simulink library "hdlNFPMathLib"  (R2019a)
settings: Solver=VariableStepAuto  StartTime=0.0  StopTime=10.0  RelTol=1e-3
libraries: simulink x3, hdlcoderNFPCast x2
settings Model: Creator=The MathWorks, Inc.  LastModifiedBy=The MathWorks, Inc.
settings DataIOCC: ReturnWorkspaceOutputs=off
settings DebuggingCC: ArithmeticOperatorsInVariantConditions=warning
settings SFSimCC: SimUseLocalCustomCode=off
settings RTWCC: RTWUseLocalCustomCode=off
settings CodeAppCC: StateflowObjectComments=on

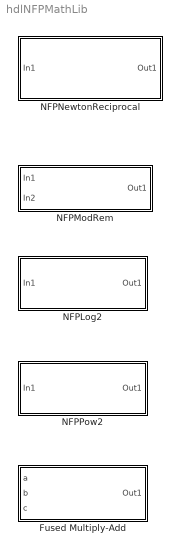
== system hdlNFPMathLib ==
  Fused Multiply-Add : Subsystem  mask(Fused Multiply-Add){FMA=on}
      mask prompts: FMA "Floating-point fused multiply-add"
      mask help: Performing fused multiply-add (FMA) operations on single inputs.
      mask init:
      | FMAstr = get_param(gcb, 'FMA');
      | if strcmp(FMAstr, 'on')
      |     fused = true;
      | else
      |     fused = false;
      | end
      mask Display:
      | port_label('input', 1, 'a');
      | port_label('input', 2, 'b');
      | port_label('input', 3, 'c');
      | 
      | FMAstr = get_param(gcb, 'FMA');
      | 
      | if strcmp(FMAstr, 'on')
      |     disp('c + (a.*b)\n\n(fused)');
      | else
      |     disp('c + (a.*b)');
      | end
  NFPLog2 : Subsystem
  NFPModRem : Subsystem  VariantControl=Variant1  mask{MAX_ITERATIONS=0, ModOrRem=Rem, MaxIterations=32, ModOrRemText=0}
      mask prompts: MAX_ITERATIONS "NumberOfIterations"; ModOrRem "Function"
      mask init:
      | if (ModOrRem == 1)
      |     ModOrRemText = 'Rem';
      | else
      |     ModOrRemText = 'Mod';
      | end
      | 
      | if (MaxIterations == 1)
      |     MAX_ITERATIONS = 32;
      | elseif (MaxIterations == 2)
      |     MAX_ITERATIONS = 64;
      | else
      |     MAX_ITERATIONS = 128;
      | end
      mask TypeOptions ModOrRem: Rem | Mod
      mask TypeOptions MaxIterations: 32 | 64 | 128
      mask Display: disp(ModOrRemText)
  NFPNewtonReciprocal : Subsystem  mask(NFP Newton Raphson Reciprocal){NumberOfIterations=3, SampleTime=-1}
      mask prompts: NumberOfIterations "Number Of Iterations"
      mask help:
      | For floating-point datatype, this block uses fixed-point arithmetics in each NR iteration while 'HDL Reciprocal' block uses floating-point arithmetics.
      |
      | Fixed-point datatype is not supported with this block.
      mask init:
      | numIters = NumberOfIterations;
  NFPPow2 : Subsystem

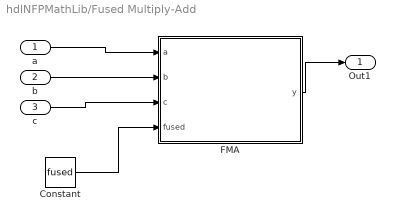
== system hdlNFPMathLib/Fused Multiply-Add ==
  a : Inport
  b : Inport  Port=2
  c : Inport  Port=3
  Constant : Constant  Value=fused  SampleTime=-1
  FMA : MATLAB Function  TreatAsAtomicUnit=on  mask{Function=0}
      mask init:
      | Function = 'pow2';
  Out1 : Outport
  wires:
  a/1 -> FMA/1(a)
  FMA/1(y) -> Out1/1
  b/1 -> FMA/2(b)
  c/1 -> FMA/3(c)
  Constant/1 -> FMA/4(fused)

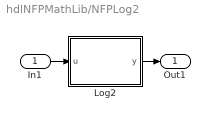
== system hdlNFPMathLib/NFPLog2 ==
  In1 : Inport
  Log2 : MATLAB Function  TreatAsAtomicUnit=on  mask{Function=0}
      mask init:
      | Function = 'log2';
  Out1 : Outport
  wires:
  In1/1 -> Log2/1(u)
  Log2/1(y) -> Out1/1

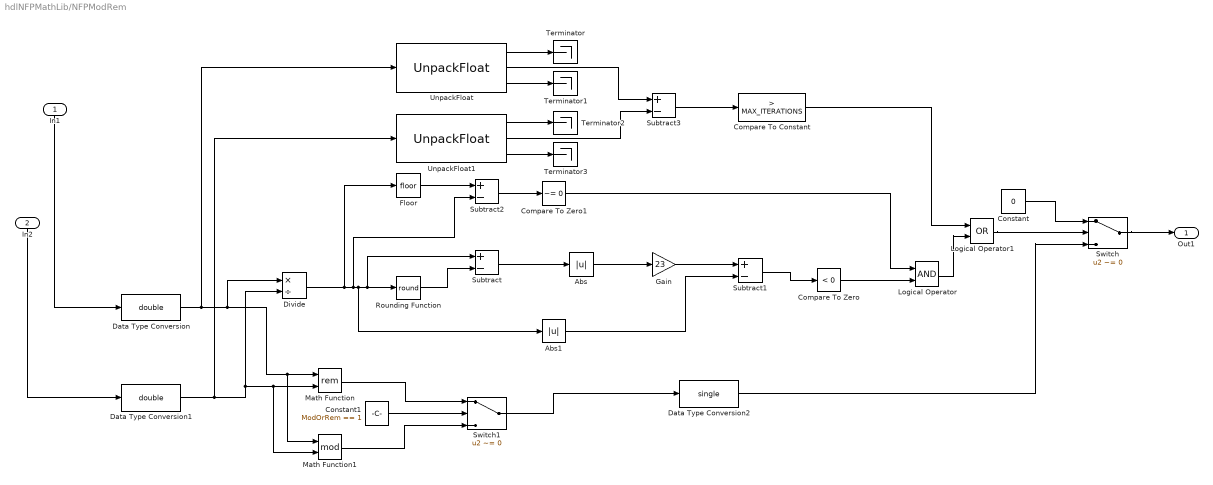
== system hdlNFPMathLib/NFPModRem ==
  In1 : Inport
  In2 : Inport  Port=2
  Abs : Abs
  Abs1 : Abs
  Compare To Constant : simulink/Logic and Bit Operations/Compare To Constant  relop=>  const=MAX_ITERATIONS  OutDataTypeStr=boolean
  Compare To Zero : simulink/Logic and Bit Operations/Compare To Zero  relop=<  OutDataTypeStr=boolean
  Compare To Zero1 : simulink/Logic and Bit Operations/Compare To Zero  relop=~=  OutDataTypeStr=boolean
  Constant : Constant  Value=0  OutDataTypeStr=single  SampleTime=-1
  Constant1 : Constant  Value=ModOrRem == 1  SampleTime=-1
  Data Type Conversion : DataTypeConversion  OutDataTypeStr=double
  Data Type Conversion1 : DataTypeConversion  OutDataTypeStr=double
  Data Type Conversion2 : DataTypeConversion  OutDataTypeStr=single
  Divide : Product  Inputs=*/  SaturateOnIntegerOverflow=on  RndMeth=Zero
  Floor : Rounding
  Gain : Gain  Gain=23
  Logical Operator : Logic  AllPortsSameDT=off  OutDataTypeStr=boolean
  Logical Operator1 : Logic  Operator=OR  AllPortsSameDT=off  OutDataTypeStr=boolean
  Math Function : Math  Operator=rem  SaturateOnIntegerOverflow=on
  Math Function1 : Math  Operator=mod  SaturateOnIntegerOverflow=on
  Rounding Function : Rounding  Operator=round
  Subtract : Sum  Inputs=+-
  Subtract1 : Sum  Inputs=+-
  Subtract2 : Sum  Inputs=+-
  Subtract3 : Sum  Inputs=+-  AccumDataTypeStr=int16  OutDataTypeStr=int16  SaturateOnIntegerOverflow=on
  Switch : Switch  Criteria=u2 ~= 0
  Switch1 : Switch  Criteria=u2 ~= 0
  Terminator{,1..3} (4 alike) : Terminator
  UnpackFloat : hdlcoderNFPCast/UnpackFloat  dataType=double
      settings: SourceProductName=Simulink  SourceProductBaseCode=SL
  UnpackFloat1 : hdlcoderNFPCast/UnpackFloat  dataType=double
      settings: SourceProductName=Simulink  SourceProductBaseCode=SL
  Out1 : Outport
  wires:
  In1/1 -> Data Type Conversion/1
  In2/1 -> Data Type Conversion1/1
  Data Type Conversion1/1 -> UnpackFloat1/1, Math Function1/2, Math Function/2, Divide/2
  Data Type Conversion/1 -> UnpackFloat/1, Math Function1/1, Math Function/1, Divide/1
  Data Type Conversion2/1 -> Switch/3
  Subtract/1 -> Abs/1
  Rounding Function/1 -> Subtract/2
  Divide/1 -> Floor/1, Subtract2/2, Abs1/1, Subtract/1, Rounding Function/1
  Abs/1 -> Gain/1
  Gain/1 -> Subtract1/1
  Abs1/1 -> Subtract1/2
  Compare To Zero/1 -> Logical Operator/2
  Subtract1/1 -> Compare To Zero/1
  Switch/1 -> Out1/1
  Constant/1 -> Switch/1
  Floor/1 -> Subtract2/1
  Subtract2/1 -> Compare To Zero1/1
  Logical Operator1/1 -> Switch/2
  Compare To Zero1/1 -> Logical Operator/1
  UnpackFloat/1 -> Terminator/1
  UnpackFloat/3 -> Terminator1/1
  UnpackFloat1/3 -> Terminator3/1
  UnpackFloat1/1 -> Terminator2/1
  UnpackFloat/2 -> Subtract3/1
  UnpackFloat1/2 -> Subtract3/2
  Subtract3/1 -> Compare To Constant/1
  Logical Operator/1 -> Logical Operator1/2
  Compare To Constant/1 -> Logical Operator1/1
  Switch1/1 -> Data Type Conversion2/1
  Math Function1/1 -> Switch1/3
  Math Function/1 -> Switch1/1
  Constant1/1 -> Switch1/2

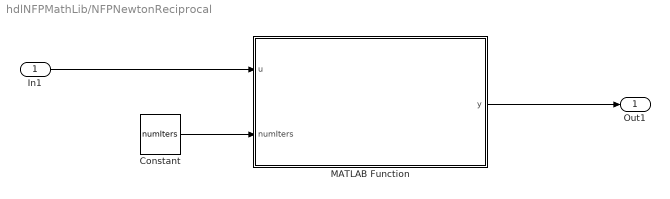
== system hdlNFPMathLib/NFPNewtonReciprocal ==
  In1 : Inport
  Constant : Constant  Value=numIters  VectorParams1D=off  OutDataTypeStr=uint8  SampleTime=-1
  MATLAB Function : MATLAB Function  TreatAsAtomicUnit=on
  Out1 : Outport
  wires:
  Constant/1 -> MATLAB Function/2(numIters)
  In1/1 -> MATLAB Function/1(u)
  MATLAB Function/1(y) -> Out1/1

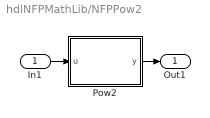
== system hdlNFPMathLib/NFPPow2 ==
  In1 : Inport
  Pow2 : MATLAB Function  TreatAsAtomicUnit=on  mask{Function=0}
      mask init:
      | Function = 'pow2';
  Out1 : Outport
  wires:
  Pow2/1(y) -> Out1/1
  In1/1 -> Pow2/1(u)

== matlab function hdlNFPMathLib/NFPLog2/Log2 ==
  data: u input; y output
function y = LOG2(u)
%#codegen
    u = double(u);
    y = zeros(size(u), 'single');
    
    for ii = 1:1:numel(u)
        if (u(ii) < 0)
            y(ii) = single(NaN);
        else
            y(ii) = single(log(u(ii))/log(2));
        end
    end
end

== matlab function hdlNFPMathLib/NFPNewtonReciprocal/MATLAB Function ==
  data: u input; y output; numIters input
function y = eml_al_nr_reciprocal_v2(u,numIters)
% Algorithm Lowering Library Function for Newto-Raphson reciprocal

% Copyright 2013-2014 MathWorks,Inc.
%#codegen

% y = 1/u

coder.allowpcode('plain');
% 
% if ~isempty(coder.target)
%     eml_prefer_const(u);
%     eml_prefer_const(numIters);
% end

%Compute input argument dimensions
sz = size(u);
if isfi(u)
    outLen = numberofelements(u);
else
    outLen = numel(u);
end

% Pre-allocation and initialization

% double input
if isa(u,'double')
    y = coder.nullcopy(zeros(sz));
    uInput = double(0);     
end

% single input
if isa(u,'single')
    y = coder.nullcopy(single(zeros(sz)));
    uInput = single(0);    
end

% fixed point input
if ~isfloat(u)
    assert('Non-floating data types are not supported');
    return;
    
    [uNT,yNT,yFm] = locaGetOutputFixptAttrib(u);
    
    if (yNT.FractionLength == 0)
        switch(yNT.WordLength)
            case 8
                if yNT.SignednessBool
                    y = int8(0);
                else
                    y = uint8(0);
                end
            case 16
                if yNT.SignednessBool
                    y = int16(0);
                else
                    y = uint16(0);
                end
            case 32
                if yNT.SignednessBool
                    y = int32(0);
                else
                    y = uint32(0);
                end
            case 64
                if yNT.SignednessBool
                    y = int64(0);
                else
                    y = uint64(0);
                end
            otherwise
                y = coder.nullcopy(fi(zeros(sz),yNT));
        end
    else
        y = coder.nullcopy(fi(zeros(sz),yNT));
    end

    uInput = fi(u,uNT,yFm);
end

% Newton-Raphson Reciprocal Algorithm
for idx = 1:outLen
    u_idx = u(idx);
    
    if (u_idx < cast(0,'like',u_idx))
        uInput(:) = -u_idx;
        u_sign_change = true;
    else
        uInput(:) = u_idx;
        u_sign_change = false;
    end
    
    % Newton-Raphson kernel iterations
    if isfloat(uInput)
        % floating point
        b = reciprocal_nr_kernel(uInput,numIters);
    else
        % fixed point
        b = reciprocal_nr_kernel_fi(uInput,numIters);
    end
    
    if u_sign_change
        y(idx) = -b;
    else
        y(idx) = b;
    end
    
end

end   % function

% ------------------------------------------
% local function
% ------------------------------------------
function b  = reciprocal_nr_kernel(a,n)
% kernel to iteratively compute Newton-Raphson reciprocal
%#codegen
% 
% if ~isempty(coder.target)
%     eml_prefer_const(n);
% end

if a == cast(0,'like',a)
    b = cast(1/a,'like',a);
    return;
elseif abs(a) == cast(inf,'like',a)    
    b = cast(1/a,'like',a);    
    return;
end

f = abs(a);

[t,e] = log2(f);

b = cast(1,'like',a);

if ~isfloat(a) || isnan(a)
    for i = 1:n
        b(:) =  b*(2-b*t);
    end
else
    if strcmpi('single', class(a))
        MWL = 25; MFL = 23;
    else % double
        MWL = 25; MFL = 23;
    end
    fm = fimath(hdlfimath, 'ProductMode', 'SpecifyPrecision', ...
        'ProductWordLength', MWL, 'ProductFractionLength', MFL, ...
        'SumMode', 'SpecifyPrecision', ...
        'SumWordLength', MWL, 'SumFractionLength', MFL);
    b = fi(b, 0, MWL, MFL, fm);
    t = fi(t, 0, MWL, MFL, fm);
    x = fi(2, 0, MWL, MFL, fm);
    for i = 1:n
        b(:) =  b*(x-b*t);
    end
    b = cast(b, 'like', a);
end

b = b*pow2(-e);

end

% -----------------------------------------
% fixed-point kernel
% -----------------------------------------
function y = reciprocal_nr_kernel_fi(u,n)
%# codegen 

[a,p] = fxpFREXP(u);

isInputZero = isequal(u,cast(0,'like',u));

% if input is zero, no need to denormalize result
% since it is the max value for the output format

if isInputZero && (p > cast(0,'like',p))
    p = cast(0,'like',p);
end

localFm = u.fimath;

wl = u.WordLength;
fl = u.FractionLength;

b = fi(1,0,wl,wl-2,localFm);

for i = 1:n
    b(:) = b*(cast(2,'like',b) - b*a); 
end

if u.Signed
    extraIntLength = 1;
else
    extraIntLength = 0;
end

output_fl = (wl-fl-1-extraIntLength);

if b.WordLength > 1   
    if p >= 0  
        if isInputZero
            b = bitsra(b,extraIntLength);
        end
        
        keep_extra_bit = 1-fl-extraIntLength;    % Extra number of LSB to keep
                                                 % (before being thrown away by bitsra()),
                                                 % which is distance between fractionlength of 
                                                 % intermediate datatype and
                                                 % output datatype, which
                                                 % is equal to [output_fl - (wl-2)] 
        
        if ((keep_extra_bit >0) && ~isInputZero)
            y = reinterpretcast(bitsra(b,p-1),numerictype(false,wl,wl-1)); % keep one extra bit to have better precision
            y = fi(y,numerictype(u.Signed,wl,output_fl));
        else
            y = fi(bitsra(b,p),numerictype(u.Signed,wl,output_fl));
        end
    else
        b = reinterpretcast(b,numerictype(false,wl,0));
        y = reinterpretcast(bitsra(b,fl-1+p),numerictype(false,wl,wl-fl-1));
        y = fi(y,numerictype(u.Signed,wl,output_fl));
    end
else
    y = b;
    y = fi(y,numerictype(u.Signed,wl,output_fl));
end

end

% ----------------------------------------
% fixed point normalization function
% ----------------------------------------
function [y,r]= fxpFREXP(u)
% fxpFREXP(u): Range normalization for fixed-point
%
% This function assumes:
%
%   1) u is a POSITIVE-valued
%   2) u is a FI fixed-point binary point scaled type
%   3) 2 < u.WordLength <= 128
%
% *** The CALLER must check for this before calling fxpFREXP ***
%# codegen 

if ~isfi(u)
    error('fi:internal:mustbefi','Input must be fi.\n');
end

WL = u.WordLength;

if WL > 128
    error('fi:internal:mustlessthan128','Word Length of fi object cannot exceed 128\n');
end

if WL == 1
    v = reinterpretcast(fi(u,false,2,u.FractionLength),numerictype(false,2,0));
else
    v = reinterpretcast(u,numerictype(false,WL,0));
end

if WL > 64
    % Assuming 64< WL <= 128 
    
    % NOTE: (2^64 - 1) not representable in a double with 52-bit mantissa
    r  = bitsll(int16(v > fi(2^64-1,false,WL,0,'hex','ffffffffffffffff')), 6);
    v  = bitsra(v, r);

    sh = bitsll(int16(v > (2^32 - 1)), 5);
    v  = bitsra(v, sh);
    r  = bitor( r, sh);

    sh = bitsll(int16(v > (2^16 - 1)), 4);
    v  = bitsra(v, sh);
    r  = bitor( r, sh);

    sh = bitsll(int16(v > ( 2^8 - 1)), 3);
    v  = bitsra(v, sh);
    r  = bitor( r, sh);

    sh = bitsll(int16(v > ( 2^4 - 1)), 2);
    v  = bitsra(v, sh);
    r  = bitor( r, sh);

    sh = bitsll(int16(v > ( 2^2 - 1)), 1);
    v  = bitsra(v, sh);
    r  = bitor( r, sh);
    
    elseif WL > 32
    % Assuming 32 < WL <= 64 here
    r  = bitsll(int16(v > (2^32 - 1)), 5);
    v  = bitsra(v, r);

    sh = bitsll(int16(v > (2^16 - 1)), 4);
    v  = bitsra(v, sh);
    r  = bitor( r, sh);

    sh = bitsll(int16(v > ( 2^8 - 1)), 3);
    v  = bitsra(v, sh);
    r  = bitor( r, sh);

    sh = bitsll(int16(v > ( 2^4 - 1)), 2);
    v  = bitsra(v, sh);
    r  = bitor( r, sh);

    sh = bitsll(int16(v > ( 2^2 - 1)), 1);
    v  = bitsra(v, sh);
    r  = bitor( r, sh);
    
elseif WL > 16
    % Assuming 16 < WL <= 32 here
    r  = bitsll(int16(v > (2^16 - 1)), 4);
    v  = bitsra(v, r);

    sh = bitsll(int16(v > ( 2^8 - 1)), 3);
    v  = bitsra(v, sh);
    r  = bitor( r, sh);

    sh = bitsll(int16(v > ( 2^4 - 1)), 2);
    v  = bitsra(v, sh);
    r  = bitor( r, sh);

    sh = bitsll(int16(v > ( 2^2 - 1)), 1);
    v  = bitsra(v, sh);
    r  = bitor( r, sh);
    
elseif WL > 8
    % Assuming 8 < WL <= 16 here
    r  = bitsll(int16(v > ( 2^8 - 1)), 3);
    v  = bitsra(v, r);

    sh = bitsll(int16(v > ( 2^4 - 1)), 2);
    v  = bitsra(v, sh);
    r  = bitor( r, sh);

    sh = bitsll(int16(v > ( 2^2 - 1)), 1);
    v  = bitsra(v, sh);
    r  = bitor( r, sh);
    
else
    % Assuming 4 < WL <= 8 here
    r  = bitsll(int16(v > ( 2^4 - 1)), 2);
    v  = bitsra(v, r);

    sh = bitsll(int16(v > ( 2^2 - 1)), 1);
    v  = bitsra(v, sh);
    r  = bitor( r, sh);
end

r = bitor( r, bitsra(int16(v),1) ) + 1;  % plus one for ceiling

r = r - cast(u.FractionLength,'like',r); % signed integer value

if u.WordLength > 1
    y = reinterpretcast(bitsll(u,WL-u.FractionLength-r),numerictype(false,WL,WL));
else
    y = reinterpretcast(u,numerictype(false,WL,WL));
end

end % function

% ----------------------------------
% Helper function to get fixedpoint attribute by internal rule
% localGetOutputFixptAttrbs(u)
% ----------------------------------
function [uNT,yNT,yFm] = locaGetOutputFixptAttrib(u)

if ~isempty(coder.target)
    eml_prefer_const(u);
end

if isinteger(u)
    switch class(u)
        case 'int8'
            uWL =  8; isUnsUInput = 0;
        case 'uint8'
            uWL =  8; isUnsUInput = 1;
        case 'int16'
            uWL = 16; isUnsUInput = 0;
        case 'uint16'
            uWL = 16; isUnsUInput = 1;
        case 'int32'
            uWL = 32; isUnsUInput = 0;
        case 'uint32'
            uWL = 32; isUnsUInput = 1;
        case 'int64'
            uWL = 64; isUnsUInput = 0;
        otherwise
            uWL = 64; isUnsUInput = 1;
    end
    uFL = 0;
else
    % Assuming U is a FI type
    isUnsUInput = double((~isfloat(u)) && (~issigned(u)));
    uNT         = eml_al_numerictype(u);
    uWL         = uNT.WordLength;
    uFL         = uNT.FractionLength;
end

if isUnsUInput
    extraIntLength = 1;
else
    extraIntLength = 2;
end

if isfi(u) && isscaleddouble(u)
    uNT = numerictype(...
        'Signed',     ~isUnsUInput,...
        'WordLength',     uWL,...
        'FractionLength', uFL,...
        'DataTypeMode',   'Scaled double: binary point scaling');
    yNT = numerictype(...
        'Signed',     ~isUnsUInput,...
        'WordLength',     uWL,...
        'FractionLength', uWL-uFL-extraIntLength,...
        'DataTypeMode',   'Scaled double: binary point scaling');
else
    uNT = numerictype(~isUnsUInput, uWL, uFL);
    yNT = numerictype(~isUnsUInput, uWL, uWL-uFL-extraIntLength);
end

yFm = fimath(...
    'ProductMode',           'SpecifyPrecision', ...
    'ProductWordLength',     uWL, ...
    'ProductFractionLength', uWL-2,...
    'SumMode',               'SpecifyPrecision', ...
    'SumWordLength',         uWL, ...
    'SumFractionLength',     uWL-2,...
    'RoundMode',             'Floor', ...
    'OverflowMode',          'Saturate'...
    );

end % function

% [EOF]

== matlab function hdlNFPMathLib/NFPPow2/Pow2 ==
  data: u input; y output
function y = POW2(u)
%#codegen
    u = single(u);
    y = zeros(size(u), 'single');
    
    for ii = 1:1:numel(u)
        y(ii) = pow2(u(ii));
    end
end

== matlab function hdlNFPMathLib/Fused Multiply-Add/FMA ==
  data: a input; y output; b input; c input; fused input
function y = FMA(a, b, c, fused)
%#codegen
    a = single(a);
    b = single(b);
    c = single(c);
    
    a_cf = CustomFloat(a);
    b_cf = CustomFloat(b);
    c_cf = CustomFloat(c);
    
    if (fused)
        y_cf = fma(a_cf, b_cf, c_cf);
    else
        y_cf = (a_cf .* b_cf) + c_cf;
    end
    
    y = single(y_cf);
end
